simulink model "HSat_orbit"  (R2023a)
settings: Solver=FixedStepAuto  StartTime=0  StopTime=86400*900  MaxStep=3600  RelTol=1e-3  EnableMultiTasking=on
values from neighbouring files (symbols this model uses):
  ext_ENV_G = 6.674e-11    [HSat_op_setup.m]    (also in HSat_op_setup_merged_maria.m)
  ext_ENV_muEarth = 3.986005e14    (= 398600500000000)    [GEO_insertion_setup.m]    (also in HSat_op_setup.m; HSat_op_setup_merged_maria.m; init_orbit_analysis_with_drag_loss.m)
  ext_ENV_Re = 6.37813700*10^6    (= 6378137)    [HSat_op_setup.m]    (also in HSat_op_setup_merged_maria.m)
  ext_EOR_atmosphere_end = 1000e3    (= 1000000)    [HSat_op_setup.m]    (also in HSat_op_setup_merged_maria.m)
  ext_EOR_perigeeraise_end = 600e3    (= 600000)    [HSat_op_setup.m]    (also in HSat_op_setup_merged_maria.m)
  ext_Main_initDate_IC_T = sim_start    [HSat_op_setup.m]    (also in HSat_op_setup_merged_maria.m)
  ext_SC_activecorr_COE_ECI = [1, 1, 1, 0, 0, 0, 0, 0 ]    [HSat_op_setup.m]    (also in HSat_op_setup_merged_maria.m)
  ext_SC_balanced_COE_ECI = [ .500    0.70    1.100 1 1]    [HSat_op_setup.m]    (also in HSat_op_setup_merged_maria.m = [ 0.10 2.10 1.40    1.0000    1.0000]; launch_settings.m)
  ext_SC_cutofferror_COE_ECI = [150e3, .01, 0.1*pi/180, .1*pi/180,.1*pi/180, 0, 0, 0]    [HSat_op_setup.m]    (also in HSat_op_setup_merged_maria.m)
  ext_SC_init_COE_ECI = [a0,ecc0,i0,an0,ap0,tran0,eccan0,ma0]    [HSat_op_setup.m]    (also in HSat_op_setup_merged_maria.m)
  ext_SC_target_COE_ECI = [a1,ecc1,i1,an1,ap1,tran1,eccan1,ma1]    [HSat_op_setup.m]    (also in HSat_op_setup_merged_maria.m)
  ext_SC_target_lambda = 67*pi/180    (= 1.16937059884)    [HSat_op_setup.m]    (also in HSat_op_setup_merged_maria.m)
  sim_SC_init_CoG_EOR_dry = [-0.00448 0.00106 0.46931]    [HSat_op_setup.m]    (also in HSat_op_setup_merged_maria.m)
  sim_SC_init_CoG_propellant = [0 0 0.24758]    [HSat_op_setup.m]    (also in HSat_op_setup_merged_maria.m)
  sim_SC_init_dry_mass = sim_SC_init_wet_mass-sim_SC_init_propellant_mass    (= 727)    [HSat_op_setup.m]    (also in HSat_op_setup_merged_maria.m = 813.7)
  sim_SC_init_wet_mass = 750    [HSat_op_setup.m]    (also in HSat_op_setup_merged_maria.m)
  sim_thrust_force = [ ... (first row only)    [HSat_op_setup.m]    (also in HSat_op_setup_merged_maria.m)
  sim_thrust_massflow = [ ... (first row only)    [HSat_op_setup.m]    (also in HSat_op_setup_merged_maria.m)
  sim_thrust_vector = [ ... (first row only)    [HSat_op_setup.m]    (also in HSat_op_setup_merged_maria.m)
  sim_thruster_position = [ ... (first row only)    [HSat_op_setup.m]    (also in HSat_op_setup_merged_maria.m)
  sim_ts_save = 60    [HSat_op_setup.m]    (also in HSat_op_setup_merged_maria.m)
  third_body_jupiter = 1    [HSat_op_setup.m]    (also in HSat_op_setup_merged_maria.m)
  third_body_moon = 1    [HSat_op_setup.m]    (also in HSat_op_setup_merged_maria.m)
  third_body_sun = 1    [HSat_op_setup.m]    (also in HSat_op_setup_merged_maria.m)
libraries: aerolibutil x26, simulink x12, sharedtransform x7, sharedutil x4, Toolbox x3, matrix_library x1, simulink_extras x1
(part 1 of 5)
settings Model: Creator=EVI  LastModifiedBy=mariahoflund
settings SolverCC: AlgebraicLoopSolver=TrustRegion
settings DataIOCC: LimitDataPoints=on  SaveFormat=Array  SignalLoggingSaveFormat=ModelDataLogs  ReturnWorkspaceOutputs=off
settings OptimizationCC: ReuseModelBlockBuffer=off  ExpressionDepthLimit=2147483647  InitFltsAndDblsToZero=on  LifeSpan=inf
settings DebuggingCC: SaveWithParameterizedLinksMsg=none  UnderspecifiedInitializationDetection=Classic  MergeDetectMultiDrivingBlocksExec=none  SignalResolutionControl=TryResolveAllWithWarning  SolverPrmCheckMsg=warning  MultiTaskDSMMsg=warning  MultiTaskCondExecSysMsg=none  FcnCallInpInsideContextMsg=warning  UnconnectedInputMsg=warning  UnconnectedOutputMsg=warning  UnconnectedLineMsg=warning  StateNameClashWarn=warning  SFUnexpectedBacktrackingDiag=warning  SFNoUnconditionalDefaultTransitionDiag=warning  SFExecutionAtInitializationDiag=none  ArithmeticOperatorsInVariantConditions=warning
settings HardwareCC: ProdBitPerPointer=32  ProdBitPerSizeT=32  ProdBitPerPtrDiffT=32  ProdLargestAtomicFloat=None  ProdIntDivRoundTo=Undefined  ProdEndianess=Unspecified  ProdWordSize=32  ProdHWDeviceType=32-bit Generic
settings ModelReferenceCC: EnableRefExpFcnMdlSchedulingChecks=on  PropagateSignalLabelsOutOfModel=off
settings SFSimCC: SimParseCustomCode=off
settings RTWCC: DLArmComputeVersion=19.05
settings CodeAppCC: StateflowObjectComments=on
settings GRTTargetCC: TargetFcnLib=ansi_tfl_tmw.mat  TargetLangStandard=C89/C90 (ANSI)  CombineOutputUpdateFcns=off  GRTInterface=on
settings ConfigComp: CovMetricSettings=dw  CovSaveCumulativeToWorkspaceVar=on  CovSaveSingleToWorkspaceVar=on

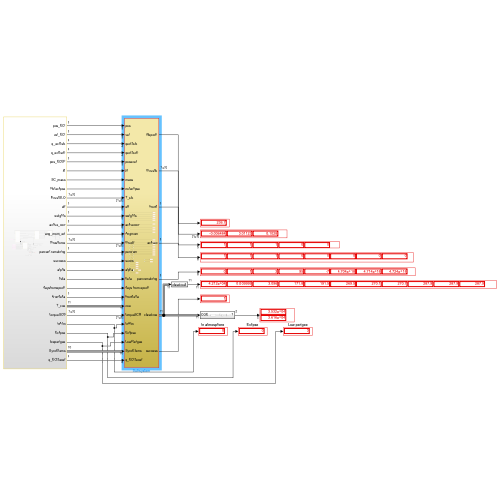
[thumbnail: Simulink's stored preview of the top-level diagram]
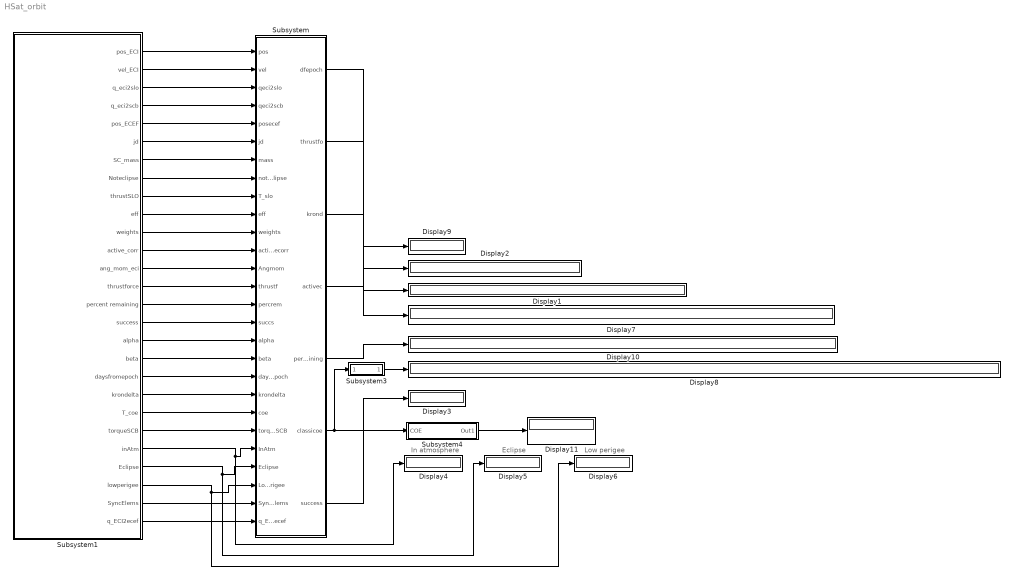
== system HSat_orbit ==
  note: Low perigee
  note: Eclipse
  note: In atmosphere
  Display{1..11} (11 alike) : Display
  Subsystem : Subsystem
  Subsystem1 : Subsystem
  Subsystem3 : Subsystem
  Subsystem4 : Subsystem
  wires:
  Subsystem3/1(Out1) -> Display8/1
  Subsystem1/20(krondelta) -> Subsystem/20(krondelta)
  Subsystem1/21(T_coe) -> Subsystem/21(coe)
  Subsystem1/12(active_corr) -> Subsystem/12(activecorr)
  Subsystem1/1(pos_ECI) -> Subsystem/1(pos)
  Subsystem1/2(vel_ECI) -> Subsystem/2(vel)
  Subsystem1/3(q_eci2slo) -> Subsystem/3(qeci2slo)
  Subsystem1/4(q_eci2scb) -> Subsystem/4(qeci2scb)
  Subsystem1/5(pos_ECEF) -> Subsystem/5(posecef)
  Subsystem1/6(jd) -> Subsystem/6(jd)
  Subsystem1/7(SC_mass) -> Subsystem/7(mass)
  Subsystem1/8(Noteclipse) -> Subsystem/8(noteclipse)
  Subsystem1/10(eff) -> Subsystem/10(eff)
  Subsystem1/11(weights) -> Subsystem/11(weights)
  Subsystem/3(krond) -> Display1/1
  Subsystem/4(activec) -> Display7/1
  Subsystem/6(classicoe) -> Subsystem3/1(classicoe), Subsystem4/1(COE)
  Subsystem1/19(daysfromepoch) -> Subsystem/19(days from epoch)
  Subsystem1/14(thrustforce) -> Subsystem/14(thrustf)
  Subsystem/2(thrustfo) -> Display2/1
  Subsystem/1(dfepoch) -> Display9/1
  Subsystem1/15(percent remaining) -> Subsystem/15(percrem)
  Subsystem/5(percremaining) -> Display10/1
  Subsystem/7(success) -> Display3/1
  Subsystem1/16(success) -> Subsystem/16(succs)
  Subsystem1/17(alpha) -> Subsystem/17(alpha)
  Subsystem1/18(beta) -> Subsystem/18(beta)
  Subsystem1/13(ang_mom_eci) -> Subsystem/13(Angmom)
  Subsystem1/9(thrustSLO) -> Subsystem/9(T_slo)
  Subsystem1/22(torqueSCB) -> Subsystem/22(torqueSCB)
  Subsystem1/23(inAtm) -> Display4/1, Subsystem/23(InAtm)
  Subsystem1/24(Eclipse) -> Display5/1, Subsystem/24(Eclipse)
  Subsystem1/25(lowperigee) -> Display6/1, Subsystem/25(LowPerigee)
  Subsystem4/1(Out1) -> Display11/1
  Subsystem1/26(SyncElems) -> Subsystem/26(SyncElems)
  Subsystem1/27(q_ECI2ecef) -> Subsystem/27(q_ECI2ecef)

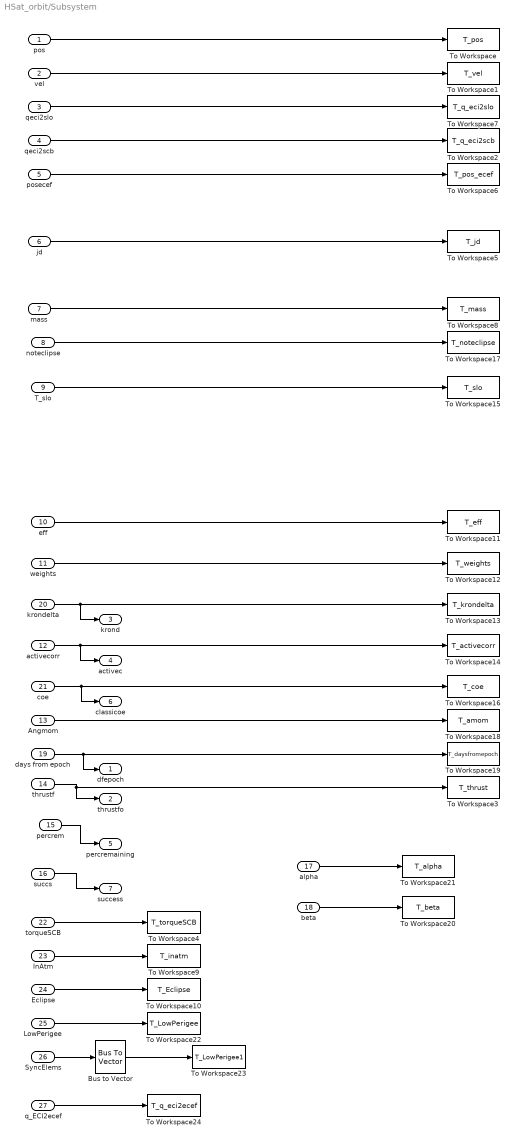
== system HSat_orbit/Subsystem ==
  pos : Inport
  vel : Inport  Port=2
  qeci2slo : Inport  Port=3
  qeci2scb : Inport  Port=4
  posecef : Inport  Port=5
  jd : Inport  Port=6
  mass : Inport  Port=7
  noteclipse : Inport  Port=8
  T_slo : Inport  Port=9
  eff : Inport  Port=10
  weights : Inport  Port=11
  activecorr : Inport  Port=12
  Angmom : Inport  Port=13
  thrustf : Inport  Port=14
  percrem : Inport  Port=15
  succs : Inport  Port=16
  alpha : Inport  Port=17
  beta : Inport  Port=18
  days from epoch : Inport  Port=19
  krondelta : Inport  Port=20
  coe : Inport  Port=21
  torqueSCB : Inport  Port=22
  InAtm : Inport  Port=23
  Eclipse : Inport  Port=24
  LowPerigee : Inport  Port=25
  SyncElems : Inport  Port=26
  q_ECI2ecef : Inport  Port=27
  Bus to Vector : BusToVector
  To Workspace : ToWorkspace  VariableName=T_pos  SampleTime=sim_ts_save
  To Workspace1 : ToWorkspace  VariableName=T_vel  SampleTime=sim_ts_save
  To Workspace10 : ToWorkspace  VariableName=T_Eclipse  SampleTime=sim_ts_save
      settings: Save2DSignal=2-D array (concatenate along first dimension)
  To Workspace11 : ToWorkspace  VariableName=T_eff  SampleTime=sim_ts_save
  To Workspace12 : ToWorkspace  VariableName=T_weights  SampleTime=sim_ts_save
  To Workspace13 : ToWorkspace  VariableName=T_krondelta  SampleTime=sim_ts_save
  To Workspace14 : ToWorkspace  VariableName=T_activecorr  SampleTime=sim_ts_save
  To Workspace15 : ToWorkspace  VariableName=T_slo  SampleTime=sim_ts_save
      settings: Save2DSignal=2-D array (concatenate along first dimension)
  To Workspace16 : ToWorkspace  VariableName=T_coe  SampleTime=sim_ts_save
  To Workspace17 : ToWorkspace  VariableName=T_noteclipse  SampleTime=sim_ts_save
  To Workspace18 : ToWorkspace  VariableName=T_amom  SampleTime=sim_ts_save
      settings: Save2DSignal=2-D array (concatenate along first dimension)
  To Workspace19 : ToWorkspace  VariableName=T_daysfromepoch  SampleTime=sim_ts_save
      settings: Save2DSignal=2-D array (concatenate along first dimension)
  To Workspace2 : ToWorkspace  VariableName=T_q_eci2scb  SampleTime=sim_ts_save
  To Workspace20 : ToWorkspace  VariableName=T_beta  SampleTime=sim_ts_save
  To Workspace21 : ToWorkspace  VariableName=T_alpha  SampleTime=sim_ts_save
  To Workspace22 : ToWorkspace  VariableName=T_LowPerigee  SampleTime=sim_ts_save
      settings: Save2DSignal=2-D array (concatenate along first dimension)
  To Workspace23 : ToWorkspace  VariableName=T_LowPerigee1  SampleTime=sim_ts_save
      settings: Save2DSignal=2-D array (concatenate along first dimension)
  To Workspace24 : ToWorkspace  VariableName=T_q_eci2ecef  SampleTime=sim_ts_save
      settings: Save2DSignal=2-D array (concatenate along first dimension)
  To Workspace3 : ToWorkspace  VariableName=T_thrust  SampleTime=sim_ts_save
      settings: Save2DSignal=2-D array (concatenate along first dimension)
  To Workspace4 : ToWorkspace  VariableName=T_torqueSCB  SampleTime=sim_ts_save
      settings: Save2DSignal=2-D array (concatenate along first dimension)
  To Workspace5 : ToWorkspace  VariableName=T_jd  SampleTime=sim_ts_save
  To Workspace6 : ToWorkspace  VariableName=T_pos_ecef  SampleTime=sim_ts_save
  To Workspace7 : ToWorkspace  VariableName=T_q_eci2slo  SampleTime=sim_ts_save
  To Workspace8 : ToWorkspace  VariableName=T_mass  SampleTime=sim_ts_save
  To Workspace9 : ToWorkspace  VariableName=T_inatm  SampleTime=sim_ts_save
      settings: Save2DSignal=2-D array (concatenate along first dimension)
  dfepoch : Outport
  thrustfo : Outport  Port=2
  krond : Outport  Port=3
  activec : Outport  Port=4
  percremaining : Outport  Port=5
  classicoe : Outport  Port=6
  success : Outport  Port=7
  wires:
  eff/1 -> To Workspace11/1
  activecorr/1 -> activec/1, To Workspace14/1
  qeci2scb/1 -> To Workspace2/1
  qeci2slo/1 -> To Workspace7/1
  posecef/1 -> To Workspace6/1
  T_slo/1 -> To Workspace15/1
  weights/1 -> To Workspace12/1
  jd/1 -> To Workspace5/1
  vel/1 -> To Workspace1/1
  pos/1 -> To Workspace/1
  noteclipse/1 -> To Workspace17/1
  mass/1 -> To Workspace8/1
  krondelta/1 -> krond/1, To Workspace13/1
  coe/1 -> classicoe/1, To Workspace16/1
  Angmom/1 -> To Workspace18/1
  days from epoch/1 -> To Workspace19/1, dfepoch/1
  thrustf/1 -> To Workspace3/1, thrustfo/1
  percrem/1 -> percremaining/1
  succs/1 -> success/1
  alpha/1 -> To Workspace21/1
  beta/1 -> To Workspace20/1
  torqueSCB/1 -> To Workspace4/1
  InAtm/1 -> To Workspace9/1
  Eclipse/1 -> To Workspace10/1
  LowPerigee/1 -> To Workspace22/1
  SyncElems/1 -> Bus to Vector/1
  Bus to Vector/1 -> To Workspace23/1
  q_ECI2ecef/1 -> To Workspace24/1

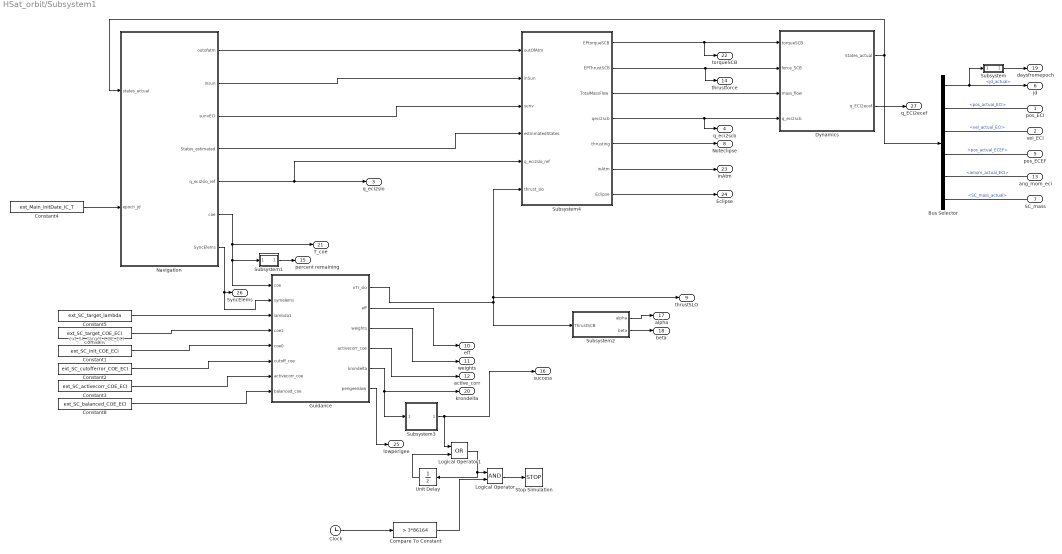
== system HSat_orbit/Subsystem1 ==
  note: ext_SC_target_COE_ECI
  Bus Selector : BusSelector  OutputSignals=jd_actual,pos_actual_ECI,vel_actual_ECI,pos_actual_ECEF,amom_actual_ECI,SC_mass_actual
  Clock : Clock
  Compare To Constant : simulink/Logic and Bit Operations/Compare To Constant  relop=>  const=3*86164  OutDataTypeStr=boolean
  Constant : Constant  Value=ext_SC_target_COE_ECI
  Constant1 : Constant  Value=ext_SC_init_COE_ECI
  Constant2 : Constant  Value=ext_SC_cutofferror_COE_ECI
  Constant3 : Constant  Value=ext_SC_activecorr_COE_ECI
  Constant4 : Constant  Value=ext_Main_initDate_IC_T
  Constant5 : Constant  Value=ext_SC_target_lambda
  Constant8 : Constant  Value=ext_SC_balanced_COE_ECI
  Dynamics : Subsystem
  Guidance : Subsystem
  Logical Operator : Logic  AllPortsSameDT=off  OutDataTypeStr=boolean
  Logical Operator1 : Logic  Operator=OR  AllPortsSameDT=off  OutDataTypeStr=boolean
  Navigation : Subsystem
  Stop Simulation : Stop
  Subsystem : Subsystem
  Subsystem1 : Subsystem
  Subsystem2 : Subsystem
  Subsystem3 : Subsystem
  Subsystem4 : Subsystem
  Unit Delay : UnitDelay  SampleTime=-1  HasFrameUpgradeWarning=on
  pos_ECI : Outport
  vel_ECI : Outport  Port=2
  q_eci2slo : Outport  Port=3
  q_eci2scb : Outport  Port=4
  pos_ECEF : Outport  Port=5
  jd : Outport  Port=6
  SC_mass : Outport  Port=7
  Noteclipse : Outport  Port=8
  thrustSLO : Outport  Port=9
  eff : Outport  Port=10
  weights : Outport  Port=11
  active_corr : Outport  Port=12
  ang_mom_eci : Outport  Port=13
  thrustforce : Outport  Port=14
  percent remaining : Outport  Port=15
  success : Outport  Port=16
  alpha : Outport  Port=17
  beta : Outport  Port=18
  daysfromepoch : Outport  Port=19
  krondelta : Outport  Port=20
  T_coe : Outport  Port=21
  torqueSCB : Outport  Port=22
  inAtm : Outport  Port=23
  Eclipse : Outport  Port=24
  lowperigee : Outport  Port=25
  SyncElems : Outport  Port=26
  q_ECI2ecef : Outport  Port=27
  wires:
  Bus Selector/2 -> pos_ECI/1  "<pos_actual_ECI>"
  Bus Selector/3 -> vel_ECI/1  "<vel_actual_ECI>"
  Bus Selector/6 -> SC_mass/1  "<SC_mass_actual>"
  Bus Selector/4 -> pos_ECEF/1  "<pos_actual_ECEF>"
  Subsystem/1(Out1) -> daysfromepoch/1
  Subsystem1/1(Out1) -> percent remaining/1
  Subsystem3/1(success) -> success/1, Logical Operator1/1
  Bus Selector/5 -> ang_mom_eci/1  "<amom_actual_ECI>"
  Bus Selector/1 -> jd/1, Subsystem/1(In1)  "<jd_actual>"
  Guidance/5(krondelta) -> krondelta/1, Subsystem3/1(krondelta)
  Constant/1 -> Guidance/4(coe1)
  Constant1/1 -> Guidance/5(coe0)
  Constant2/1 -> Guidance/6(cutoff_coe)
  Constant3/1 -> Guidance/7("activecorr_coe ")
  Constant8/1 -> Guidance/8(balanced_coe)
  Guidance/2(eff) -> eff/1
  Guidance/3(weights) -> weights/1
  Guidance/4(activecorr_coe) -> active_corr/1
  Dynamics/1(States_actual) -> Bus Selector/1, Navigation/1(states_actual)
  Guidance/1(nTr_slo) -> Subsystem2/1(ThrustSCB), Subsystem4/6(thrust_slo), thrustSLO/1
  Navigation/5(q_eci2slo_ref) -> Subsystem4/5(q_eci2slo_ref), q_eci2slo/1
  Navigation/6(coe) -> Subsystem1/1(coe), Guidance/1(coe), T_coe/1
  Constant4/1 -> Navigation/2(epoch_jd)
  Navigation/7(SyncElems) -> Guidance/2(symelems), SyncElems/1
  Subsystem4/1(EPtorqueSCB) -> Dynamics/1(torqueSCB), torqueSCB/1
  Subsystem4/2(EPThrustSCB) -> thrustforce/1, Dynamics/2(force_SCB)
  Subsystem4/4(qeci2scb) -> Dynamics/4(q_eci2scb), q_eci2scb/1
  Navigation/1(outofatm) -> Subsystem4/1(outOfAtm)
  Navigation/2(insun) -> Subsystem4/2(inSun)
  Navigation/3(sunvECI) -> Subsystem4/3(sunv)
  Navigation/4(States_estimated) -> Subsystem4/4(estinmatedStates)
  Subsystem4/3(TotalMassFlow) -> Dynamics/3(mass_flow)
  Subsystem4/5(thrusting) -> Noteclipse/1
  Subsystem4/6(inAtm) -> inAtm/1
  Subsystem4/7(Eclipse) -> Eclipse/1
  Constant5/1 -> Guidance/3(lambda1)
  Subsystem2/2(beta) -> beta/1
  Subsystem2/1(alpha) -> alpha/1
  Guidance/6(perigeeislow) -> lowperigee/1
  Logical Operator/1 -> Stop Simulation/1
  Clock/1 -> Compare To Constant/1
  Compare To Constant/1 -> Logical Operator/2
  Logical Operator1/1 -> Unit Delay/1, Logical Operator/1
  Unit Delay/1 -> Logical Operator1/2
  Dynamics/2(q_ECI2ecef) -> q_ECI2ecef/1

== system HSat_orbit/Subsystem3 ==
  classicoe : Inport
  Demux4 : Demux  Outputs=11
  Gain : Gain  Gain=1e-3
  Mux : Mux  Inputs=11
  Subsystem : Subsystem
  Subsystem1 : Subsystem
  Subsystem2 : Subsystem
  Subsystem3 : Subsystem
  Subsystem4 : Subsystem
  Subsystem5 : Subsystem
  Subsystem6 : Subsystem
  Subsystem7 : Subsystem
  Subsystem8 : Subsystem
  Out1 : Outport
  wires:
  classicoe/1 -> Demux4/1
  Mux/1 -> Out1/1
  Demux4/1 -> Gain/1
  Gain/1 -> Mux/1
  Demux4/2 -> Mux/2
  Demux4/3 -> Subsystem/1(In1)
  Demux4/5 -> Subsystem2/1(In1)
  Demux4/7 -> Subsystem4/1(In1)
  Demux4/9 -> Subsystem6/1(In1)
  Demux4/11 -> Subsystem8/1(In1)
  Subsystem/1(Out1) -> Mux/3
  Demux4/4 -> Subsystem1/1(In1)
  Demux4/6 -> Subsystem3/1(In1)
  Demux4/8 -> Subsystem5/1(In1)
  Demux4/10 -> Subsystem7/1(In1)
  Subsystem1/1(Out1) -> Mux/4
  Subsystem2/1(Out1) -> Mux/5
  Subsystem3/1(Out1) -> Mux/6
  Subsystem4/1(Out1) -> Mux/7
  Subsystem5/1(Out1) -> Mux/8
  Subsystem6/1(Out1) -> Mux/9
  Subsystem7/1(Out1) -> Mux/10
  Subsystem8/1(Out1) -> Mux/11

== system HSat_orbit/Subsystem4 ==
  COE : Inport
  Gain : Gain  Gain=1e-3
  Gain1 : Gain  Gain=1e-3
  Mux : Mux  Inputs=2
  Subsystem2 : Subsystem
  Out1 : Outport
  wires:
  Gain/1 -> Mux/1
  COE/1 -> Subsystem2/1(COE)
  Gain1/1 -> Mux/2
  Subsystem2/1(Perigee altitude) -> Gain/1
  Subsystem2/2(Apogee altitude) -> Gain1/1
  Mux/1 -> Out1/1

== system HSat_orbit/Subsystem1/Dynamics ==
  torqueSCB : Inport
  force_SCB : Inport  Port=2
  mass_flow : Inport  Port=3
  q_eci2scb : Inport  Port=4
  Bus Creator : BusCreator  Inputs=7
  Integrator : Integrator
  Integrator1 : Integrator
  Quaternion Inverse1 : aerolibutil/Quaternion Inverse
  Quaternion Rotation : aerolibutil/Quaternion Rotation
  Subsystem : Subsystem
  Sum : Sum  Inputs=|-+
  sim_Target_mass : Constant  Value=sim_SC_init_wet_mass
  States_actual : Outport
  q_ECI2ecef : Outport  Port=2
  wires:
  force_SCB/1 -> Subsystem/2(SC_thrust_force_SCB)
  Subsystem/4(pos_ECEF) -> Bus Creator/5  "pos_actual_ECEF"
  sim_Target_mass/1 -> Sum/2
  mass_flow/1 -> Integrator/1
  Integrator/1 -> Sum/1
  Sum/1 -> Subsystem/3(SC_mass), Bus Creator/6  "SC_mass_actual"
  Subsystem/3(vicrf) -> Bus Creator/4  "vel_actual_ECI"
  Subsystem/1(jd) -> Bus Creator/2  "jd_actual"
  Quaternion Rotation/1 -> Integrator1/1
  Integrator1/1 -> Bus Creator/1  "amom_actual_ECI"
  torqueSCB/1 -> Quaternion Rotation/2
  Quaternion Inverse1/1 -> Quaternion Rotation/1
  q_eci2scb/1 -> Quaternion Inverse1/1, Bus Creator/7, Subsystem/1(SC_attitude_eci2scb)  "q_eci2scb"
  Bus Creator/1 -> States_actual/1
  Subsystem/2(xicrf) -> Bus Creator/3  "pos_actual_ECI"
  Subsystem/5(q_ECI2ecef) -> q_ECI2ecef/1

== system HSat_orbit/Subsystem1/Guidance ==
  coe : Inport
  symelems : Inport  Port=2
  lambda1 : Inport  Port=3
  coe1 : Inport  Port=4
  coe0 : Inport  Port=5
  cutoff_coe : Inport  Port=6
  "activecorr_coe " : Inport  Port=7
  balanced_coe : Inport  Port=8
  Bus Creator : BusCreator  Inputs=5
  Bus Selector : BusSelector  OutputSignals=nT_transfer_slo,eff,weights,krondelta,activecorr_coe
  Bus to Vector : BusToVector
  MATLAB Function1 : MATLAB Function  TreatAsAtomicUnit=on
  Subsystem1 : Subsystem
  nTr_slo : Outport
  eff : Outport  Port=2
  weights : Outport  Port=3
  activecorr_coe : Outport  Port=4
  krondelta : Outport  Port=5
  perigeeislow : Outport  Port=6
  wires:
  MATLAB Function1/4(krondelta) -> Bus Creator/4  "krondelta"
  MATLAB Function1/5(activecorr_coe) -> Bus Creator/5  "activecorr_coe"
  MATLAB Function1/2(eff) -> Bus Creator/2  "eff"
  MATLAB Function1/1(nT_slo) -> Bus Creator/1  "nT_transfer_slo"
  MATLAB Function1/3(weights) -> Bus Creator/3  "weights"
  Bus Creator/1 -> Bus Selector/1
  Bus Selector/1 -> nTr_slo/1  "<nT_transfer_slo>"
  Bus Selector/2 -> eff/1  "<eff>"
  Bus Selector/3 -> weights/1  "<weights>"
  Bus Selector/4 -> krondelta/1  "<krondelta>"
  Bus Selector/5 -> activecorr_coe/1  "<activecorr_coe>"
  coe/1 -> Subsystem1/1(coe)
  symelems/1 -> Subsystem1/2(symelems)
  lambda1/1 -> Subsystem1/3(lambda1)
  coe1/1 -> Subsystem1/4(coe1)
  coe0/1 -> Subsystem1/5(coe0)
  cutoff_coe/1 -> Subsystem1/6(cutoff_coe)
  "activecorr_coe "/1 -> Subsystem1/7("activecorr_coe ")
  balanced_coe/1 -> Subsystem1/8(balanced_coe)
  Subsystem1/1(COE) -> Bus to Vector/1
  Subsystem1/2(Coe1Out) -> MATLAB Function1/2(coe1)
  Subsystem1/3(COE0Out) -> MATLAB Function1/3(coe0)
  Subsystem1/4(CutOff_COE) -> MATLAB Function1/4(cutoff_coe)
  Subsystem1/5(ActiveCOEOut) -> MATLAB Function1/5("activecorr_coe ")
  Subsystem1/6(BalancedCOE Out) -> MATLAB Function1/6(balanced_coe)
  Subsystem1/7(perigeeislow) -> perigeeislow/1
  Bus to Vector/1 -> MATLAB Function1/1(coe)

== system HSat_orbit/Subsystem1/Navigation ==
  states_actual : Inport
  epoch_jd : Inport  Port=2
  Bus Creator : BusCreator  Inputs=7
  Bus Selector : BusSelector  OutputSignals=jd_actual,pos_actual_ECI,vel_actual_ECI,pos_actual_ECEF,amom_actual_ECI,SC_mass_actual,q_eci2scb
  Bus Selector2 : BusSelector  OutputSignals=jd_actual,pos_actual_ECI,vel_actual_ECI
  Subsystem : Subsystem
  Subsystem7 : Subsystem
  Subsystem8 : Subsystem
  q_slo : Subsystem
  outofatm : Outport
  insun : Outport  Port=2
  sunvECI : Outport  Port=3
  States_estimated : Outport  Port=4
  q_eci2slo_ref : Outport  Port=5
  coe : Outport  Port=6
  SyncElems : Outport  Port=7
  wires:
  Subsystem7/1(outofatm) -> outofatm/1
  Bus Selector2/3 -> q_slo/2(velECI)  "<vel_actual_ECI>"
  q_slo/1(qECI2slo) -> q_eci2slo_ref/1  "q_eci2slo_ref"
  Bus Creator/1 -> Bus Selector2/1, States_estimated/1
  Bus Selector2/1 -> Subsystem8/1(Julian Date)  "<jd_actual>"
  Subsystem8/1(insun) -> insun/1
  Subsystem8/2(sunvECI) -> sunvECI/1
  Bus Selector2/2 -> q_slo/1(posECI), Subsystem8/2(X_icrf), Subsystem7/1(scpos)  "<pos_actual_ECI>"
  Bus Selector/6 -> Bus Creator/6  "<SC_mass_actual>"
  Bus Selector/5 -> Bus Creator/5  "<amom_actual_ECI>"
  Bus Selector/4 -> Bus Creator/4  "<pos_actual_ECEF>"
  Bus Selector/3 -> Bus Creator/3, Subsystem/4(<vel_actual_ECI>)  "<vel_actual_ECI>"
  Bus Selector/2 -> Subsystem/3(<pos_actual_ECI>), Bus Creator/2  "<pos_actual_ECI>"
  Bus Selector/1 -> Subsystem/2(<jd_actual>), Bus Creator/1  "<jd_actual>"
  states_actual/1 -> Bus Selector/1
  epoch_jd/1 -> Subsystem/1(epoch_jd)
  Subsystem/1(SyncElems) -> SyncElems/1
  Subsystem/2(coe) -> coe/1
  Bus Selector/7 -> Bus Creator/7  "<q_eci2scb>"

== system HSat_orbit/Subsystem1/Subsystem ==
  In1 : Inport
  Constant4 : Constant  Value=ext_Main_initDate_IC_T
  Floor : Rounding
  Gain : Gain  Gain=100
  Gain1 : Gain  Gain=.01
  Sum1 : Sum  Inputs=|+-
  Out1 : Outport
  wires:
  Gain1/1 -> Out1/1
  Gain/1 -> Floor/1
  Constant4/1 -> Sum1/2
  Floor/1 -> Gain1/1
  In1/1 -> Sum1/1
  Sum1/1 -> Gain/1

== system HSat_orbit/Subsystem1/Subsystem1 ==
  coe : Inport
  Add : Sum  Inputs=+-
  Add1 : Sum  Inputs=+-
  Bus Selector : BusSelector  OutputSignals=sms,ecc,incl,raan,argp,truean,eccan,meanan
  Constant5 : Constant  Value=ext_SC_target_COE_ECI
  Constant6 : Constant  Value=ext_SC_init_COE_ECI
  Constant7 : Constant  Value=ext_SC_target_COE_ECI
  Divide : Product  Inputs=*/
  Floor1 : Rounding
  Gain2 : Gain  Gain=100
  Mux : Mux  Inputs=8
  Out1 : Outport
  wires:
  Add1/1 -> Divide/1
  Add/1 -> Divide/2
  Constant5/1 -> Add/1
  Constant7/1 -> Add1/1
  Gain2/1 -> Floor1/1
  Constant6/1 -> Add/2
  Divide/1 -> Gain2/1
  Floor1/1 -> Out1/1
  coe/1 -> Bus Selector/1
  Bus Selector/1 -> Mux/1  "<sms>"
  Bus Selector/2 -> Mux/2  "<ecc>"
  Bus Selector/3 -> Mux/3  "<incl>"
  Bus Selector/4 -> Mux/4  "<raan>"
  Bus Selector/5 -> Mux/5  "<argp>"
  Bus Selector/6 -> Mux/6  "<truean>"
  Bus Selector/7 -> Mux/7  "<eccan>"
  Bus Selector/8 -> Mux/8  "<meanan>"
  Mux/1 -> Add1/2

== system HSat_orbit/Subsystem1/Subsystem2 ==
  note: [alpha,beta]=cart2sph(nT_slo(:,1),-nT_slo(:,2),-nT_slo(:,3));
      | alpha=-alpha;
  ThrustSCB : Inport
  Cartesian to Spherical : simulink_extras/Transformations/Cartesian to Spherical
  Constant : Constant  Value=pi/2
  Demux : Demux  Outputs=3
  Sum : Sum  Inputs=|-+
  Terminator : Terminator
  Unary Minus : UnaryMinus
  Unary Minus1 : UnaryMinus
  Unary Minus2 : UnaryMinus
  alpha : Outport
  beta : Outport  Port=2
  wires:
  Unary Minus2/1 -> alpha/1
  Cartesian to Spherical/2 -> Unary Minus2/1
  Demux/1 -> Cartesian to Spherical/1
  Cartesian to Spherical/1 -> Terminator/1
  Sum/1 -> beta/1
  Constant/1 -> Sum/2
  Unary Minus1/1 -> Cartesian to Spherical/3
  Unary Minus/1 -> Cartesian to Spherical/2
  Demux/3 -> Unary Minus1/1
  Cartesian to Spherical/3 -> Sum/1
  ThrustSCB/1 -> Demux/1
  Demux/2 -> Unary Minus/1

== system HSat_orbit/Subsystem1/Subsystem3 ==
  krondelta : Inport
  Demux : Demux  Outputs=5
  Logical Operator : Logic  Inputs=3  AllPortsSameDT=off  OutDataTypeStr=boolean
  Mux : Mux  Inputs=2
  Terminator : Terminator
  success : Outport
  wires:
  Mux/1 -> Terminator/1
  Demux/2 -> Logical Operator/2
  Logical Operator/1 -> success/1
  Demux/4 -> Mux/1
  krondelta/1 -> Demux/1
  Demux/5 -> Mux/2
  Demux/3 -> Logical Operator/3
  Demux/1 -> Logical Operator/1

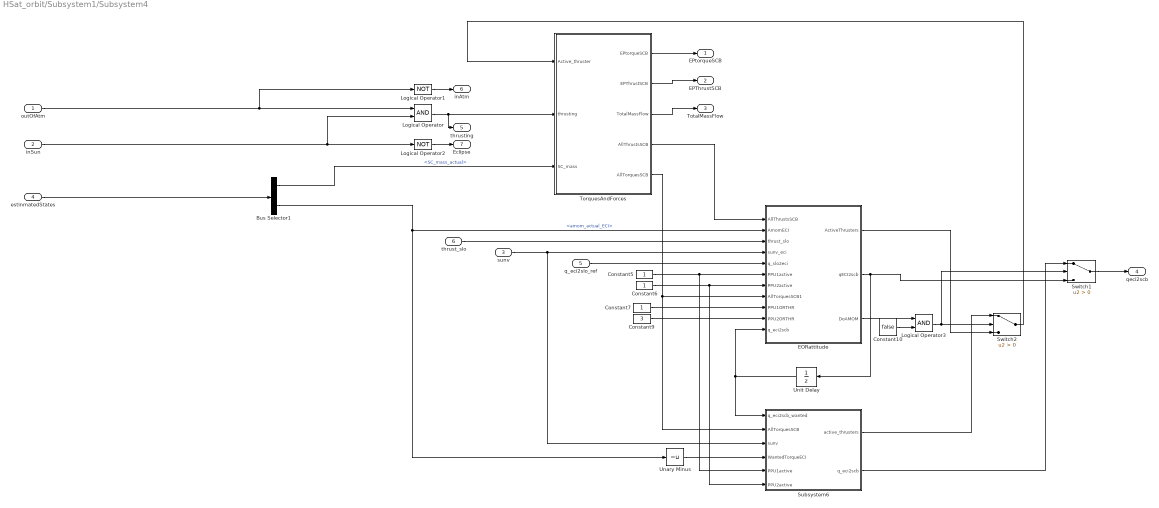
== system HSat_orbit/Subsystem1/Subsystem4 ==
  outOfAtm : Inport
  inSun : Inport  Port=2
  sunv : Inport  Port=3
  estinmatedStates : Inport  Port=4
  q_eci2slo_ref : Inport  Port=5
  thrust_slo : Inport  Port=6
  Bus Selector1 : BusSelector  OutputSignals=SC_mass_actual,amom_actual_ECI
  Constant10 : Constant  Value=false
  Constant5 : Constant
  Constant6 : Constant
  Constant7 : Constant
  Constant9 : Constant  Value=3
  EORattitude : Subsystem
  Logical Operator : Logic  AllPortsSameDT=off  OutDataTypeStr=boolean
  Logical Operator1 : Logic  Operator=NOT  AllPortsSameDT=off  OutDataTypeStr=boolean
  Logical Operator2 : Logic  Operator=NOT  AllPortsSameDT=off  OutDataTypeStr=boolean
  Logical Operator3 : Logic  AllPortsSameDT=off  OutDataTypeStr=boolean
  Subsystem6 : Subsystem
  Switch1 : Switch  Criteria=u2 > Threshold  SaturateOnIntegerOverflow=off  InputSameDT=off
  Switch2 : Switch  Criteria=u2 > Threshold  SaturateOnIntegerOverflow=off  InputSameDT=off
  TorquesAndForces : Subsystem
  Unary Minus : UnaryMinus
  Unit Delay : UnitDelay  InitialCondition=[1 0 0 0]  SampleTime=-1  HasFrameUpgradeWarning=on
  EPtorqueSCB : Outport
  EPThrustSCB : Outport  Port=2
  TotalMassFlow : Outport  Port=3
  qeci2scb : Outport  Port=4
  thrusting : Outport  Port=5
  inAtm : Outport  Port=6
  Eclipse : Outport  Port=7
  wires:
  Subsystem6/2(q_eci2scb) -> Switch1/1
  Logical Operator3/1 -> Switch1/2, Switch2/2
  Switch1/1 -> qeci2scb/1
  TorquesAndForces/3(TotalMassFlow) -> TotalMassFlow/1
  Logical Operator1/1 -> inAtm/1
  TorquesAndForces/1(EPtorqueSCB) -> EPtorqueSCB/1
  TorquesAndForces/2(EPThrustSCB) -> EPThrustSCB/1
  Logical Operator2/1 -> Eclipse/1
  Logical Operator/1 -> thrusting/1, TorquesAndForces/2(thrusting)
  EORattitude/2(qECI2scb) -> Unit Delay/1, Switch1/3
  Constant5/1 -> EORattitude/6(PPU1active), Subsystem6/5(PPU1active)
  q_eci2slo_ref/1 -> EORattitude/5(q_slo2eci)
  TorquesAndForces/5(AllTorquesSCB) -> Subsystem6/2(AllTorquesSCB), EORattitude/8(AllTorquesSCB1)
  Switch2/1 -> TorquesAndForces/1(Active_thruster)
  Constant9/1 -> EORattitude/10(PPU2ORTHR)
  Bus Selector1/2 -> Unary Minus/1, EORattitude/2(AmomECI)  "<amom_actual_ECI>"
  EORattitude/1(ActiveThrusters) -> Switch2/3
  outOfAtm/1 -> Logical Operator1/1, Logical Operator/1
  Constant10/1 -> Logical Operator3/2
  Constant7/1 -> EORattitude/9(PPU1ORTHR)
  Subsystem6/1(active_thrusters) -> Switch2/1
  sunv/1 -> Subsystem6/3(sunv), EORattitude/4(sunv_eci)
  inSun/1 -> Logical Operator/2, Logical Operator2/1
  Bus Selector1/1 -> TorquesAndForces/3(SC_mass)  "<SC_mass_actual>"
  Constant6/1 -> Subsystem6/6(PPU2active), EORattitude/7(PPU2active)
  Unit Delay/1 -> Subsystem6/1(q_eci2scb_wanted), EORattitude/11(q_eci2scb)
  EORattitude/3(DoAMOM) -> Logical Operator3/1
  estinmatedStates/1 -> Bus Selector1/1
  TorquesAndForces/4(AllThrustsSCB) -> EORattitude/1(AllThrustsSCB)
  Unary Minus/1 -> Subsystem6/4(WantedTorqueECI)
  thrust_slo/1 -> EORattitude/3(thrust_slo)

== system HSat_orbit/Subsystem3/Subsystem ==
  In1 : Inport
  Constant : Constant  Value=360
  Gain1 : Gain  Gain=180/pi
  Math Function : Math  Operator=mod
  Out1 : Outport
  wires:
  In1/1 -> Gain1/1
  Math Function/1 -> Out1/1
  Constant/1 -> Math Function/2
  Gain1/1 -> Math Function/1

== system HSat_orbit/Subsystem3/Subsystem1 ==
  In1 : Inport
  Constant : Constant  Value=360
  Gain1 : Gain  Gain=180/pi
  Math Function : Math  Operator=mod
  Out1 : Outport
  wires:
  In1/1 -> Gain1/1
  Math Function/1 -> Out1/1
  Constant/1 -> Math Function/2
  Gain1/1 -> Math Function/1

== system HSat_orbit/Subsystem3/Subsystem2 ==
  In1 : Inport
  Constant : Constant  Value=360
  Gain1 : Gain  Gain=180/pi
  Math Function : Math  Operator=mod
  Out1 : Outport
  wires:
  In1/1 -> Gain1/1
  Math Function/1 -> Out1/1
  Constant/1 -> Math Function/2
  Gain1/1 -> Math Function/1

== system HSat_orbit/Subsystem3/Subsystem3 ==
  In1 : Inport
  Constant : Constant  Value=360
  Gain1 : Gain  Gain=180/pi
  Math Function : Math  Operator=mod
  Out1 : Outport
  wires:
  In1/1 -> Gain1/1
  Math Function/1 -> Out1/1
  Constant/1 -> Math Function/2
  Gain1/1 -> Math Function/1

== system HSat_orbit/Subsystem3/Subsystem4 ==
  In1 : Inport
  Constant : Constant  Value=360
  Gain1 : Gain  Gain=180/pi
  Math Function : Math  Operator=mod
  Out1 : Outport
  wires:
  In1/1 -> Gain1/1
  Math Function/1 -> Out1/1
  Constant/1 -> Math Function/2
  Gain1/1 -> Math Function/1

== system HSat_orbit/Subsystem3/Subsystem5 ==
  In1 : Inport
  Constant : Constant  Value=360
  Gain1 : Gain  Gain=180/pi
  Math Function : Math  Operator=mod
  Out1 : Outport
  wires:
  In1/1 -> Gain1/1
  Math Function/1 -> Out1/1
  Constant/1 -> Math Function/2
  Gain1/1 -> Math Function/1

== system HSat_orbit/Subsystem3/Subsystem6 ==
  In1 : Inport
  Constant : Constant  Value=360
  Gain1 : Gain  Gain=180/pi
  Math Function : Math  Operator=mod
  Out1 : Outport
  wires:
  In1/1 -> Gain1/1
  Math Function/1 -> Out1/1
  Constant/1 -> Math Function/2
  Gain1/1 -> Math Function/1

== system HSat_orbit/Subsystem3/Subsystem7 ==
  In1 : Inport
  Constant : Constant  Value=360
  Gain1 : Gain  Gain=180/pi
  Math Function : Math  Operator=mod
  Out1 : Outport
  wires:
  In1/1 -> Gain1/1
  Math Function/1 -> Out1/1
  Constant/1 -> Math Function/2
  Gain1/1 -> Math Function/1

== system HSat_orbit/Subsystem3/Subsystem8 ==
  In1 : Inport
  Constant : Constant  Value=360
  Gain1 : Gain  Gain=180/pi
  Math Function : Math  Operator=mod
  Out1 : Outport
  wires:
  In1/1 -> Gain1/1
  Math Function/1 -> Out1/1
  Constant/1 -> Math Function/2
  Gain1/1 -> Math Function/1

== system HSat_orbit/Subsystem4/Subsystem2 ==
  COE : Inport
  Constant : Constant
  Constant1 : Constant  Value=ext_ENV_Re
  Demux : Demux  Outputs=2
  Product : Product
  Product1 : Product
  Selector : Selector  InputPortWidth=11  IndexOptions=Index vector (dialog)  Indices=[1 2]  OutputSizes=1
  Sum : Sum  Inputs=|-+
  Sum1 : Sum  Inputs=|++
  Sum2 : Sum  Inputs=|+-
  Sum3 : Sum  Inputs=|+-
  Perigee altitude : Outport
  Apogee altitude : Outport  Port=2
  wires:
  Product1/1 -> Sum3/1
  COE/1 -> Selector/1
  Sum1/1 -> Product1/2
  Product/1 -> Sum2/1
  Demux/2 -> Sum1/1, Sum/1
  Constant/1 -> Sum/2, Sum1/2
  Selector/1 -> Demux/1
  Sum/1 -> Product/2
  Demux/1 -> Product1/1, Product/1
  Sum2/1 -> Perigee altitude/1
  Sum3/1 -> Apogee altitude/1
  Constant1/1 -> Sum2/2, Sum3/2

== system HSat_orbit/Subsystem1/Dynamics/Subsystem ==
  SC_attitude_eci2scb : Inport
  SC_thrust_force_SCB : Inport  Port=2
  SC_mass : Inport  Port=3
  3 body perturbation legendre polynomial : Subsystem
  Add : Sum
  Divide : Product  Inputs=*/
  Ephemeris : Subsystem
      settings: PortSchema="{\"entries\":[{\"content\":{\"sides\":[{\"content\":{\"connectorIds\":[\"Out1\",\"Out2\",\"Out3\"]},\"type\":\"ConnectorPlacement.EquallySpacedRectSide\",\"uuid\":\"e633fcf3-0477-4ff0-a81d-4455c68815fb\"},{\"content\":{\"connectorIds\":[\"In1\"],\"side\":\"RIGHT\"},\"type\":\"ConnectorPlacement.EquallySpacedRectSide\",\"uuid\":\"e19e3365-4d80-4524-a5d7-f4214f0f2988\"},{\"content\":{\"side\":\"TOP\"},\"type\":\"ConnectorPlacement.EquallySpacedRectSide\",\"uuid\":\"a3adb7cc-79c0-421a-aab6-26119d48c80d\"}]},\"type\":\"ConnectorPlacement.EquallySpacedConnector\",\"uuid\":\"987b98a1-bb11-4f5a-8767-775a43bc92c1\"}],\"packageUris\":[\"http://schema.mathworks.com/mf0/Connector/R2020b\"],\"version\":\"1.0\"}"
  Gain : Gain
  Orbit Propagator Numerical (high precision) : OrbitPropagator  propagator=Numerical (high precision)  accelIn=on  startDate=ext_Main_initDate_IC_T  massSrc=Port  stateFormatNum=ICRF state vector  stateFormatKep=ICRF state vector  inertialPosition=ext_SC_init_pos_ECI  inertialVelocity=ext_SC_init_vel_ECI  fixedPosition=[-4142689.0 -2676864.7 -4669861.6]  fixedVelocity=[1452.7 -6720.7 2568.1]  gravityModel=Point-mass  customR=3396200  customMu=4.305e13  customJ2=1.0826269e-03  customOmega=4.06125949e-3  useEOPs=off  outputTransform=on  angleUnits=Radians
  Quaternion Inverse : aerolibutil/Quaternion Inverse
  Quaternion Rotation : aerolibutil/Quaternion Rotation
  Quaternion Rotation1 : aerolibutil/Quaternion Rotation
  Unit Delay : UnitDelay  SampleTime=-1  HasFrameUpgradeWarning=on
  jd : Outport
  xicrf : Outport  Port=2
  vicrf : Outport  Port=3
  pos_ECEF : Outport  Port=4
  q_ECI2ecef : Outport  Port=5
  wires:
  Quaternion Rotation/1 -> Divide/1
  SC_attitude_eci2scb/1 -> Quaternion Inverse/1  "qECI2SCB"
  Orbit Propagator Numerical (high precision)/2 -> vicrf/1  "velocity_ECI"
  SC_thrust_force_SCB/1 -> Quaternion Rotation/2
  Divide/1 -> Gain/1
  Gain/1 -> Add/1
  SC_mass/1 -> Divide/2
  Quaternion Inverse/1 -> Quaternion Rotation/1
  Orbit Propagator Numerical (high precision)/3 -> q_ECI2ecef/1, Quaternion Rotation1/1
  Quaternion Rotation1/1 -> pos_ECEF/1
  Ephemeris/2(lunar_X) -> 3 body perturbation legendre polynomial/3(r_moon)
  Orbit Propagator Numerical (high precision)/1 -> Quaternion Rotation1/2, 3 body perturbation legendre polynomial/1(r_sat), xicrf/1  "position_ECI"
  Ephemeris/3(jupiter_X) -> 3 body perturbation legendre polynomial/4(r_jupiter)
  Ephemeris/1(solar_X) -> 3 body perturbation legendre polynomial/2(r_sun)
  Orbit Propagator Numerical (high precision)/4 -> Ephemeris/1(T JD), jd/1
  Add/1 -> Orbit Propagator Numerical (high precision)/1
  Unit Delay/1 -> Add/2
  3 body perturbation legendre polynomial/1(3rdbodyacc) -> Unit Delay/1

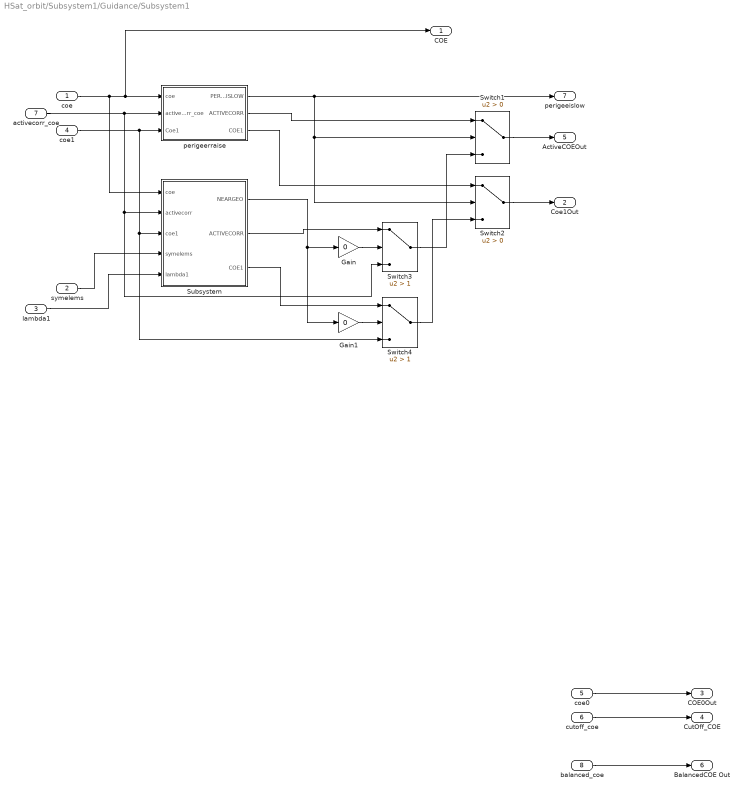
== system HSat_orbit/Subsystem1/Guidance/Subsystem1 ==
  coe : Inport
  symelems : Inport  Port=2
  lambda1 : Inport  Port=3
  coe1 : Inport  Port=4
  coe0 : Inport  Port=5
  cutoff_coe : Inport  Port=6
  "activecorr_coe " : Inport  Port=7
  balanced_coe : Inport  Port=8
  Gain : Gain  Gain=0
  Gain1 : Gain  Gain=0
  Subsystem : Subsystem
  Switch1 : Switch  Criteria=u2 > Threshold  SaturateOnIntegerOverflow=off  InputSameDT=off
  Switch2 : Switch  Criteria=u2 > Threshold  SaturateOnIntegerOverflow=off  InputSameDT=off
  Switch3 : Switch  Criteria=u2 > Threshold  Threshold=1  SaturateOnIntegerOverflow=off  InputSameDT=off
  Switch4 : Switch  Criteria=u2 > Threshold  Threshold=1  SaturateOnIntegerOverflow=off  InputSameDT=off
  perigeerraise : Subsystem
  COE : Outport
  Coe1Out : Outport  Port=2
  COE0Out : Outport  Port=3
  CutOff_COE : Outport  Port=4
  ActiveCOEOut : Outport  Port=5
  BalancedCOE Out : Outport  Port=6
  perigeeislow : Outport  Port=7
  wires:
  balanced_coe/1 -> BalancedCOE Out/1
  cutoff_coe/1 -> CutOff_COE/1
  coe0/1 -> COE0Out/1
  Switch4/1 -> Switch2/3
  coe1/1 -> Switch4/3, Subsystem/3(coe1), perigeerraise/3(Coe1)
  Switch1/1 -> ActiveCOEOut/1
  coe/1 -> Subsystem/1(coe), COE/1, perigeerraise/1(coe)
  Switch2/1 -> Coe1Out/1
  perigeerraise/1(PERIGEEISLOW) -> perigeeislow/1, Switch1/2, Switch2/2
  perigeerraise/2(ACTIVECORR) -> Switch1/1
  "activecorr_coe "/1 -> Switch3/3, Subsystem/2(activecorr), perigeerraise/2("activecorr_coe ")
  perigeerraise/3(COE1) -> Switch2/1
  symelems/1 -> Subsystem/4(symelems)
  lambda1/1 -> Subsystem/5(lambda1)
  Subsystem/1(NEARGEO) -> Gain1/1, Gain/1
  Subsystem/3(COE1) -> Switch4/1
  Subsystem/2(ACTIVECORR) -> Switch3/1
  Switch3/1 -> Switch1/3
  Gain/1 -> Switch3/2
  Gain1/1 -> Switch4/2

== system HSat_orbit/Subsystem1/Navigation/Subsystem ==
  epoch_jd : Inport
  <jd_actual> : Inport  Port=2
  <pos_actual_ECI> : Inport  Port=3
  <vel_actual_ECI> : Inport  Port=4
  Subsystem : Subsystem
  Subsystem2 : Subsystem
  SyncElems : Outport
  coe : Outport  Port=2
  wires:
  <jd_actual>/1 -> Subsystem2/1(jd)
  Subsystem2/1(SyncElems) -> SyncElems/1
  epoch_jd/1 -> Subsystem2/2(epoch_jd)
  <vel_actual_ECI>/1 -> Subsystem/2(velECI), Subsystem2/4(vel_ECI)
  <pos_actual_ECI>/1 -> Subsystem/1(posECI), Subsystem2/3(pos_ECI)
  Subsystem/1(coe) -> coe/1

== system HSat_orbit/Subsystem1/Navigation/Subsystem7 ==
  scpos : Inport
  Compare To Constant : simulink/Logic and Bit Operations/Compare To Constant  relop=>  const=ext_EOR_atmosphere_end  OutDataTypeStr=boolean
  Constant : Constant  Value=ext_ENV_Re
  Dot Product : DotProduct  OutDataTypeStr=Inherit: Inherit via internal rule
  Sqrt : Sqrt
  Sum : Sum  Inputs=|+-
  outofatm : Outport
  wires:
  scpos/1 -> Dot Product/1, Dot Product/2
  Compare To Constant/1 -> outofatm/1
  Sqrt/1 -> Sum/1
  Dot Product/1 -> Sqrt/1
  Sum/1 -> Compare To Constant/1
  Constant/1 -> Sum/2

== system HSat_orbit/Subsystem1/Navigation/Subsystem8 ==
  Julian Date : Inport
  X_icrf : Inport  Port=2
  Gain : Gain  Gain=1/1000
  Planetary Ephemeris : PlanetaryEphem  target=Sun  outputVelocity=off
  Simplified Shadow Fraction : Subsystem
  insun : Outport
  sunvECI : Outport  Port=2
  wires:
  Gain/1 -> sunvECI/1, Simplified Shadow Fraction/1(x_sun_icrf)
  Simplified Shadow Fraction/1(inView) -> insun/1
  Julian Date/1 -> Planetary Ephemeris/1
  X_icrf/1 -> Simplified Shadow Fraction/2(X_icrf)
  Planetary Ephemeris/1 -> Gain/1

== system HSat_orbit/Subsystem1/Navigation/q_slo ==
  posECI : Inport
  velECI : Inport  Port=2
  Create 3x3 Matrix : sharedutil/Create 3x3 Matrix  aMode=aMode
      settings: LibrarySourceBlock=aerolibutil/Create 3x3 Matrix
  Demux : Demux  Outputs=3
  Demux1 : Demux  Outputs=3
  Demux2 : Demux  Outputs=3
  Direction Cosine Matrix to Quaternions : sharedtransform/Direction Cosine Matrix  to Quaternions  aMode=0  action=None  tolerance=eps(2)
      settings: LibrarySourceBlock=|
      | aerolibtransform2/Direction Cosine Matrix
      | to Quaternions
  Unary Minus : UnaryMinus
  VecNormalize : Subsystem
      mask Display: disp('u/||u||')
  VecNormalize1 : Subsystem
      mask Display: disp('u/||u||')
  VecNormalize2 : Subsystem
      mask Display: disp('u/||u||')
  VecNormalize3 : Subsystem
      mask Display: disp('u/||u||')
  Z x R : Subsystem  mask(Cross Product){}
      mask help: Calculates the cross product of two 3x1 vectors.
      mask Help:
      | <p>This block calculates the cross product of two 3x1 vectors, ie.</p>
      | 
      | <ul>C(1) = A(2)*B(3) - A(3)*B(2)</ul>
      | <ul>C(2) = A(3)*B(1) - A(1)*B(3)</ul>
      | <ul>C(3) = A(1)*B(2) - A(2)*B(1)</ul>
      | 
      | <p>The block inputs and output contain more than one signal as described below.</p>
      | 
      | <p><H4>Block Vector Input 1 - A</H4>
      | <ul>
      | <li>A(1)</li>
      | <li>A(2)</li>
      | <li>A(3)</li>
      | </ul>
      | </p>
      | 
      | <p><H4>Block Vector Input 2 - B</H4>
      | <ul>
      | <li>B(1)</li>
      | <li>B(2)</li>
      | <li>B(3)</li>
      | </ul>
      | </p>
      | 
      | <p><H4>Block Vector Output - Cross Product (AxB)</H4>
      | <ul>
      | <li>C(1)</li>
      | <li>C(2)</li>
      | <li>C(3)</li>
      | </ul>
      | </p>
      mask Display: disp('Cross\nProduct')
  Z x Y : Subsystem  mask(Cross Product){}
      mask help: Calculates the cross product of two 3x1 vectors.
      mask Help:
      | <p>This block calculates the cross product of two 3x1 vectors, ie.</p>
      | 
      | <ul>C(1) = A(2)*B(3) - A(3)*B(2)</ul>
      | <ul>C(2) = A(3)*B(1) - A(1)*B(3)</ul>
      | <ul>C(3) = A(1)*B(2) - A(2)*B(1)</ul>
      | 
      | <p>The block inputs and output contain more than one signal as described below.</p>
      | 
      | <p><H4>Block Vector Input 1 - A</H4>
      | <ul>
      | <li>A(1)</li>
      | <li>A(2)</li>
      | <li>A(3)</li>
      | </ul>
      | </p>
      | 
      | <p><H4>Block Vector Input 2 - B</H4>
      | <ul>
      | <li>B(1)</li>
      | <li>B(2)</li>
      | <li>B(3)</li>
      | </ul>
      | </p>
      | 
      | <p><H4>Block Vector Output - Cross Product (AxB)</H4>
      | <ul>
      | <li>C(1)</li>
      | <li>C(2)</li>
      | <li>C(3)</li>
      | </ul>
      | </p>
      mask Display: disp('Cross\nProduct')
  qECI2slo : Outport  InitialOutput=0
  wires:
  Unary Minus/1 -> Z x Y/2(b(1) b(2) b(3)), Demux2/1, Z x R/1(a(1) a(2) a(3))  "Z"
  posECI/1 -> VecNormalize3/1(In1)
  VecNormalize3/1(Out1) -> Unary Minus/1
  velECI/1 -> VecNormalize2/1(In1)
  VecNormalize2/1(Out1) -> Z x R/2(b(1) b(2) b(3))
  Z x R/1(c(1) c(2) c(3)) -> VecNormalize1/1(In1)
  VecNormalize1/1(Out1) -> Z x Y/1(a(1) a(2) a(3)), Demux1/1  "Y"
  Z x Y/1(c(1) c(2) c(3)) -> VecNormalize/1(In1)
  VecNormalize/1(Out1) -> Demux/1  "X"
  Demux/1 -> Create 3x3 Matrix/1
  Demux/2 -> Create 3x3 Matrix/2
  Demux/3 -> Create 3x3 Matrix/3
  Demux1/1 -> Create 3x3 Matrix/4
  Demux1/2 -> Create 3x3 Matrix/5
  Demux1/3 -> Create 3x3 Matrix/6
  Demux2/1 -> Create 3x3 Matrix/7
  Demux2/2 -> Create 3x3 Matrix/8
  Demux2/3 -> Create 3x3 Matrix/9
  Create 3x3 Matrix/1 -> Direction Cosine Matrix to Quaternions/1
  Direction Cosine Matrix to Quaternions/1 -> qECI2slo/1

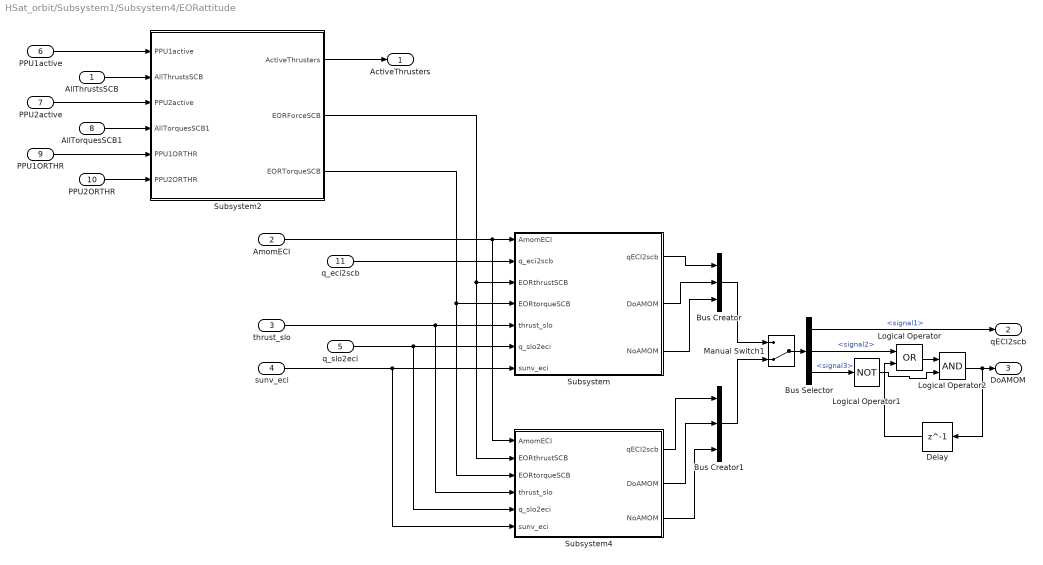
== system HSat_orbit/Subsystem1/Subsystem4/EORattitude ==
  AllThrustsSCB : Inport
  AmomECI : Inport  Port=2
  thrust_slo : Inport  Port=3
  sunv_eci : Inport  Port=4
  q_slo2eci : Inport  Port=5
  PPU1active : Inport  Port=6
  PPU2active : Inport  Port=7
  AllTorquesSCB1 : Inport  Port=8
  PPU1ORTHR : Inport  Port=9
  PPU2ORTHR : Inport  Port=10
  q_eci2scb : Inport  Port=11
  Bus Creator : BusCreator  Inputs=3
  Bus Creator1 : BusCreator  Inputs=3
  Bus Selector : BusSelector  OutputSignals=signal1,signal2,signal3
  Delay : Delay  DelayLength=1  InitialCondition=0
  Logical Operator : Logic  Operator=OR  AllPortsSameDT=off  OutDataTypeStr=boolean
  Logical Operator1 : Logic  Operator=NOT  AllPortsSameDT=off  OutDataTypeStr=boolean
  Logical Operator2 : Logic  AllPortsSameDT=off  OutDataTypeStr=boolean
  Manual Switch1 : ManualSwitch  CurrentSetting=0
  Subsystem : Subsystem
  Subsystem2 : Subsystem
  Subsystem4 : Subsystem
  ActiveThrusters : Outport
  qECI2scb : Outport  Port=2
  DoAMOM : Outport  Port=3
  wires:
  sunv_eci/1 -> Subsystem/7(sunv_eci), Subsystem4/6(sunv_eci)
  Subsystem2/3(EORTorqueSCB) -> Subsystem4/3(EORtorqueSCB), Subsystem/4(EORtorqueSCB)
  AmomECI/1 -> Subsystem4/1(AmomECI), Subsystem/1(AmomECI)
  Subsystem4/1(qECI2scb) -> Bus Creator1/1
  Subsystem2/2(EORForceSCB) -> Subsystem4/2(EORthrustSCB), Subsystem/3(EORthrustSCB)
  thrust_slo/1 -> Subsystem4/4(thrust_slo), Subsystem/5(thrust_slo)
  q_slo2eci/1 -> Subsystem4/5(q_slo2eci), Subsystem/6(q_slo2eci)
  Subsystem/1(qECI2scb) -> Bus Creator/1
  PPU1active/1 -> Subsystem2/1(PPU1active)
  AllThrustsSCB/1 -> Subsystem2/2(AllThrustsSCB)
  PPU2active/1 -> Subsystem2/3(PPU2active)
  AllTorquesSCB1/1 -> Subsystem2/4(AllTorquesSCB1)
  PPU1ORTHR/1 -> Subsystem2/5(PPU1ORTHR)
  PPU2ORTHR/1 -> Subsystem2/6(PPU2ORTHR)
  Subsystem2/1(ActiveThrusters) -> ActiveThrusters/1
  q_eci2scb/1 -> Subsystem/2(q_eci2scb)
  Subsystem4/2(DoAMOM) -> Bus Creator1/2
  Subsystem/2(DoAMOM) -> Bus Creator/2
  Bus Creator1/1 -> Manual Switch1/2
  Bus Creator/1 -> Manual Switch1/1
  Manual Switch1/1 -> Bus Selector/1
  Bus Selector/1 -> qECI2scb/1  "<signal1>"
  Bus Selector/2 -> Logical Operator/1  "<signal2>"
  Subsystem4/3(NoAMOM) -> Bus Creator1/3
  Subsystem/3(NoAMOM) -> Bus Creator/3
  Bus Selector/3 -> Logical Operator1/1  "<signal3>"
  Logical Operator1/1 -> Logical Operator2/2
  Logical Operator2/1 -> DoAMOM/1, Delay/1
  Delay/1 -> Logical Operator/2
  Logical Operator/1 -> Logical Operator2/1

== system HSat_orbit/Subsystem1/Subsystem4/Subsystem6 ==
  q_eci2scb_wanted : Inport
  AllTorquesSCB : Inport  Port=2
  sunv : Inport  Port=3
  WantedTorqueECI : Inport  Port=4
  PPU1active : Inport  Port=5
  PPU2active : Inport  Port=6
  Subsystem2 : Subsystem
  active_thrusters : Outport
  q_eci2scb : Outport  Port=2
  wires:
  AllTorquesSCB/1 -> Subsystem2/3(AllTorquesSCB)
  q_eci2scb_wanted/1 -> Subsystem2/4(q_eci2scb_wanted)
  PPU1active/1 -> Subsystem2/1(PPU1active)
  PPU2active/1 -> Subsystem2/2(PPU2active)
  WantedTorqueECI/1 -> Subsystem2/5(WantedTorqueECI)
  Subsystem2/1(ActiveThrusters) -> active_thrusters/1
  Subsystem2/2(q_eci2scb) -> q_eci2scb/1
  sunv/1 -> Subsystem2/6(sunv)

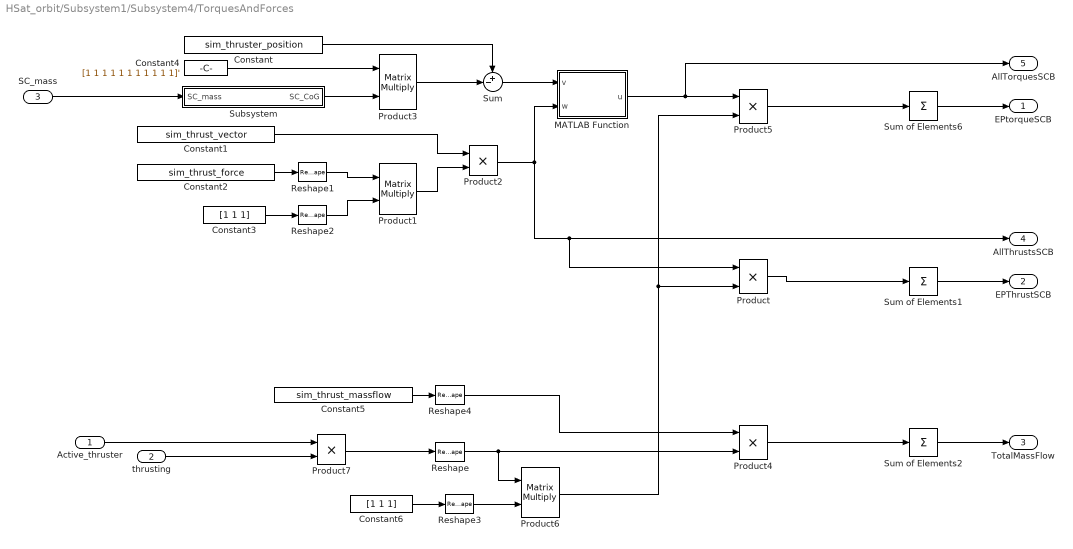
== system HSat_orbit/Subsystem1/Subsystem4/TorquesAndForces ==
  Active_thruster : Inport
  thrusting : Inport  Port=2
  SC_mass : Inport  Port=3
  Constant : Constant  Value=sim_thruster_position
  Constant1 : Constant  Value=sim_thrust_vector
  Constant2 : Constant  Value=sim_thrust_force
  Constant3 : Constant  Value=[1 1 1]
  Constant4 : Constant  Value=[1 1 1 1 1 1 1 1 1 1 1]'
  Constant5 : Constant  Value=sim_thrust_massflow
  Constant6 : Constant  Value=[1 1 1]
  MATLAB Function : MATLAB Function  TreatAsAtomicUnit=on
  Product{,2,4..5,7} (5 alike) : Product
  Product1 : Product  Multiplication=Matrix(*)
  Product3 : Product  Multiplication=Matrix(*)
  Product6 : Product  Multiplication=Matrix(*)
  Reshape : Reshape  OutputDimensionality=Column vector (2-D)
  Reshape1 : Reshape  OutputDimensionality=Column vector (2-D)
  Reshape2 : Reshape  OutputDimensionality=Row vector (2-D)
  Reshape3 : Reshape  OutputDimensionality=Row vector (2-D)
  Reshape4 : Reshape  OutputDimensionality=Column vector (2-D)
  Subsystem : Subsystem
  Sum : Sum  Inputs=+-|
  Sum of Elements1 : Sum  Inputs=+  CollapseMode=Specified dimension
  Sum of Elements2 : Sum  Inputs=+  CollapseMode=Specified dimension
  Sum of Elements6 : Sum  Inputs=+  CollapseMode=Specified dimension
  EPtorqueSCB : Outport
  EPThrustSCB : Outport  Port=2
  TotalMassFlow : Outport  Port=3
  AllThrustsSCB : Outport  Port=4
  AllTorquesSCB : Outport  Port=5
  wires:
  Sum of Elements6/1 -> EPtorqueSCB/1
  Sum of Elements1/1 -> EPThrustSCB/1
  Product5/1 -> Sum of Elements6/1
  SC_mass/1 -> Subsystem/1(SC_mass)
  Constant2/1 -> Reshape1/1
  Sum/1 -> MATLAB Function/1(v)
  Subsystem/1(SC_CoG) -> Product3/2
  Reshape1/1 -> Product1/1
  Constant1/1 -> Product2/1
  Product1/1 -> Product2/2
  Constant/1 -> Sum/1
  Constant4/1 -> Product3/1
  Constant3/1 -> Reshape2/1
  Reshape2/1 -> Product1/2
  Product3/1 -> Sum/2
  Reshape4/1 -> Product4/1
  Constant5/1 -> Reshape4/1
  Product4/1 -> Sum of Elements2/1
  Sum of Elements2/1 -> TotalMassFlow/1
  Product/1 -> Sum of Elements1/1
  MATLAB Function/1(u) -> AllTorquesSCB/1, Product5/1
  Product6/1 -> Product5/2, Product/2
  Constant6/1 -> Reshape3/1
  Reshape3/1 -> Product6/2
  Reshape/1 -> Product4/2, Product6/1
  thrusting/1 -> Product7/2
  Product7/1 -> Reshape/1
  Product2/1 -> Product/1, AllThrustsSCB/1, MATLAB Function/2(w)
  Active_thruster/1 -> Product7/1

== system HSat_orbit/Subsystem1/Dynamics/Subsystem/3 body perturbation legendre polynomial ==
  r_sat : Inport
  r_sun : Inport  Port=2
  r_moon : Inport  Port=3
  r_jupiter : Inport  Port=4
  Constant1 : Constant  Value=[0,0,0]
  Constant2 : Constant  Value=[0,0,0]
  Constant3 : Constant  Value=third_body_sun
  Constant4 : Constant  Value=third_body_moon
  Constant5 : Constant  Value=[0,0,0]
  Constant6 : Constant  Value=third_body_jupiter
  Legendre degree : Constant  Value=2
  Subsystem1 : Subsystem
  Subsystem2 : Subsystem
  Subsystem3 : Subsystem
  Subtract : Sum  Inputs=---
  Switch1 : Switch  Criteria=u2 > Threshold  SaturateOnIntegerOverflow=off  InputSameDT=off
  Switch2 : Switch  Criteria=u2 > Threshold  SaturateOnIntegerOverflow=off  InputSameDT=off
  Switch3 : Switch  Criteria=u2 > Threshold  SaturateOnIntegerOverflow=off  InputSameDT=off
  jupiter mass : Constant  Value=1.898e27
  moon mass : Constant  Value=7.342e22
  sun mass : Constant  Value=1.989e30
  3rdbodyacc : Outport
  wires:
  r_sat/1 -> Subsystem1/1(sat), Subsystem3/1(sat), Subsystem2/1(sat)
  r_sun/1 -> Subsystem2/2(3 body)
  sun mass/1 -> Subsystem2/3(mass)
  r_moon/1 -> Subsystem1/2(3 body)
  moon mass/1 -> Subsystem1/3(mass)
  r_jupiter/1 -> Subsystem3/2(3 body)
  jupiter mass/1 -> Subsystem3/3(mass)
  Subtract/1 -> 3rdbodyacc/1
  Legendre degree/1 -> Subsystem1/4(Legendre deg), Subsystem3/4(Legendre deg), Subsystem2/4(Legendre deg)
  Subsystem2/1(Out1) -> Switch1/1
  Switch1/1 -> Subtract/1
  Constant2/1 -> Switch1/3
  Constant3/1 -> Switch1/2
  Constant1/1 -> Switch2/3
  Switch2/1 -> Subtract/2
  Constant4/1 -> Switch2/2
  Subsystem1/1(Out1) -> Switch2/1
  Constant5/1 -> Switch3/3
  Switch3/1 -> Subtract/3
  Constant6/1 -> Switch3/2
  Subsystem3/1(Out1) -> Switch3/1

== system HSat_orbit/Subsystem1/Dynamics/Subsystem/Ephemeris ==
  T JD : Inport
  Gain{,1..3} (4 alike) : Gain  Gain=1000
  Jupiter Ephemeris : PlanetaryEphem  target=Jupiter
  Lunar Ephemeris : PlanetaryEphem
  Solar Ephemeris : PlanetaryEphem  target=Sun
  Terminator : Terminator
  Terminator1 : Terminator
  Terminator2 : Terminator
  km to m : Gain  Gain=1000
  km to m1 : Gain  Gain=1000
  solar_X : Outport
  lunar_X : Outport  Port=2
  jupiter_X : Outport  Port=3
  wires:
  T JD/1 -> Lunar Ephemeris/1, Jupiter Ephemeris/1, Solar Ephemeris/1
  Lunar Ephemeris/2 -> Gain1/1
  Solar Ephemeris/1 -> Gain2/1
  Solar Ephemeris/2 -> km to m/1
  Lunar Ephemeris/1 -> Gain/1
  Gain/1 -> lunar_X/1
  Gain1/1 -> Terminator2/1
  Gain2/1 -> solar_X/1
  km to m/1 -> Terminator1/1
  Jupiter Ephemeris/2 -> km to m1/1
  Gain3/1 -> jupiter_X/1
  km to m1/1 -> Terminator/1
  Jupiter Ephemeris/1 -> Gain3/1
